simulink model "airspeed_throttle"  (R2017a)
settings: Solver=VariableStepAuto  StartTime=0.0  StopTime=20  RelTol=1e-3
undefined symbols (not defined in the file): a_V1, a_V2, P
settings Model: Creator=pizzaslayer  LastModifiedBy=Parth

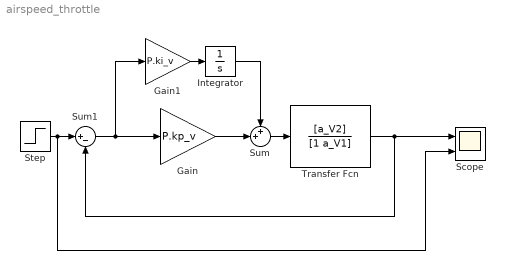
== system airspeed_throttle ==
  Gain : Gain  Gain=P.kp_v
  Gain1 : Gain  Gain=P.ki_v
  Integrator : Integrator
  Scope : Scope  NumInputPorts=2
  Step : Step  SampleTime=0
  Sum : Sum  Inputs=++|
  Sum1 : Sum  Inputs=|+-
  Transfer Fcn : TransferFcn  Numerator=[a_V2]  Denominator=[1 a_V1]
  wires:
  Gain1/1 -> Integrator/1
  Step/1 -> Scope/2, Sum1/1
  Sum1/1 -> Gain1/1, Gain/1
  Integrator/1 -> Sum/1
  Gain/1 -> Sum/2
  Transfer Fcn/1 -> Scope/1, Sum1/2
  Sum/1 -> Transfer Fcn/1
